simulink model "Exp2"  (R2020a)
settings: Solver=VariableStepAuto  StartTime=0.0  StopTime=25  RelTol=1e-3
InitFcn:
  | Voc=32.9;
  | Iscn=8.21;
  | k=1.38e-23;
  | Ns=54;
  | Np=1;
  | G=800;
  | Gn=1000;
  | Kv=-0.1230;
  | KI=0.0032;
  | T=301;
  | Tn=300;
  | q=1.6e-19;
  | n=1;
  | I0n=9.85e-8;
  | Eg=1.12;
  | Ign=8.214;
  | Rs=0.221;
  | Rp=414.5;
  | a=1.0
libraries: powerlib x7, simulink x1
settings Model: Creator=ahmed  LastModifiedBy=ahmed
settings DataIOCC: Refine=250

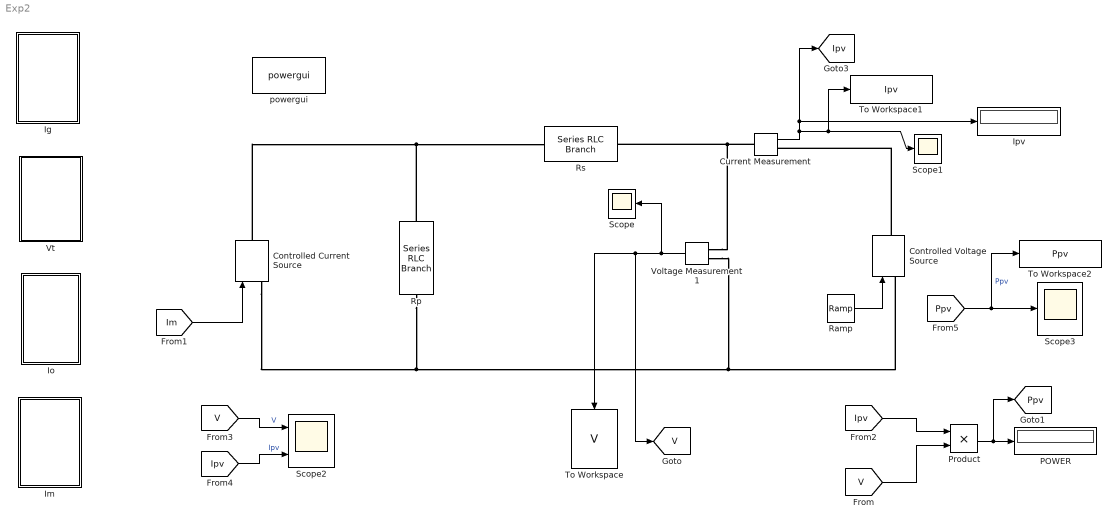
== system Exp2 ==
  Controlled Current Source : powerlib/Electrical Sources/Controlled Current Source  Initialize=on  Source_Type=AC  Amplitude=0  Phase=0  Frequency=0  Measurements=None
  Controlled Voltage Source : powerlib/Electrical Sources/Controlled Voltage Source  Initialize=on  Source_Type=AC  Amplitude=0  Phase=0  Frequency=0  Measurements=None
  Current Measurement : powerlib/Measurements/Current Measurement  PhasorSimulation=off  OutputType=Complex  PSBequivalent=0
  Ig : Subsystem
  Im : Subsystem
  Io : Subsystem
  Ipv : Display
  POWER : Display
  Product : Product
  Ramp : simulink/Sources/Ramp  slope=1  start=0  InitialOutput=0
  Rp : powerlib/Elements/Series RLC Branch  LConnTagsString=__new0  RConnTagsString=__new0  BranchType=R  Resistance=Rp  Inductance=1e-3  SetiL0=off  InitialCurrent=0  Capacitance=1e-6  Setx0=off  InitialVoltage=0  Measurements=None
  Rs : powerlib/Elements/Series RLC Branch  LConnTagsString=__new0  RConnTagsString=__new0  BranchType=R  Resistance=Rs  Inductance=1e-3  SetiL0=off  InitialCurrent=0  Capacitance=1e-6  Setx0=off  InitialVoltage=0  Measurements=None
  Scope : Scope
  Scope1 : Scope
  Scope2 : Scope  NumInputPorts=2
  Scope3 : Scope
  To Workspace : ToWorkspace  VariableName=V  SaveFormat=Timeseries  SampleTime=-1
  To Workspace1 : ToWorkspace  VariableName=Ipv  SaveFormat=Timeseries  SampleTime=-1
  To Workspace2 : ToWorkspace  VariableName=Ppv  SaveFormat=Timeseries  SampleTime=-1
  Voltage Measurement1 : powerlib/Measurements/Voltage Measurement  PhasorSimulation=off  OutputType=Complex  PSBequivalent=0
  Vt : Subsystem
  powergui : powerlib/powergui  Priority=1  SimulationMode=Continuous  SampleTime=50e-6  frequency=60  Iterations=50  frequencyindice=0  Pbase=100e6  ErrMax=1e-4  UnitsV=kV  UnitsW=MW  buscounter=0  FunctionMessages=off  echomessages=off  EnableUseOfTLC=off  CurrentSourceSwitches=off  DisableSnubberDevices=off  DisableRonSwitches=off  DisableVfSwitches=off  DisplayEquations=off  AutomaticDiscreteSolvers=off  SolverType=Tustin/Backward Euler (TBE)  Interpol=off  ExternalGateDelay=off  methode=off  Ts=100  x0status=blocks  SPID=on  SwTol=0  HookPort=off  NonlinearTolerance=1e-4  nMaxIteration=100  ContinueOnMaxIteration=off  RestoreLinks=warning  ResistiveCurrentMeasurement=off  Frange=[0:2:500]  Ylog=off  Xlog=on  ShowGrid=off  save=off  variable=ZData  structure=0  ZoomFFT=off  StartTime=0.0  cycles=1  DisplayStyle=1  fundamental=60  FreqAxis=off  MaxFrequency=1000  frequencyindicesteady=1  RmsSteady=1  display=off
  tag scope: Ipv=global, Ppv=global, V=global
  wires:
  [Im] -> Controlled Current Source/1
  Ramp/1 -> Controlled Voltage Source/1
  Voltage Measurement1/1 -> [V], To Workspace/1, Scope/1
  [Ipv] -> Product/1
  [V] -> Product/2
  Product/1 -> [Ppv], POWER/1
  [V] -> Scope2/1  "V"
  [Ipv] -> Scope2/2  "Ipv"
  [Ppv] -> To Workspace2/1, Scope3/1  "Ppv"
  Current Measurement/1 -> Scope1/1, To Workspace1/1, Ipv/1, [Ipv]
  connections:
  Controlled Current Source/RConn1 -- Rs/LConn1 -- Rp/LConn1
  Current Measurement/LConn1 -- Voltage Measurement1/LConn1 -- Rs/RConn1
  Controlled Voltage Source/RConn1 -- Current Measurement/RConn1
  Controlled Current Source/LConn1 -- Voltage Measurement1/LConn2 -- Controlled Voltage Source/LConn1 -- Rp/RConn1

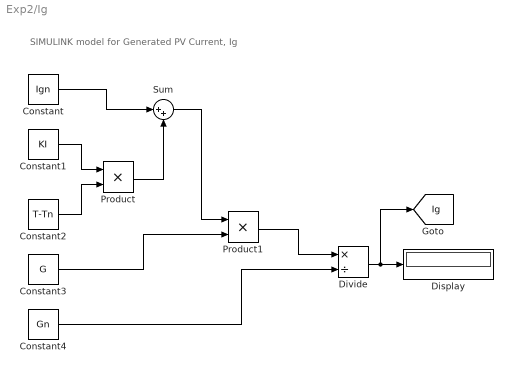
== system Exp2/Ig ==
  note: SIMULINK model for Generated PV Current, Ig
  Constant : Constant  Value=Ign
  Constant1 : Constant  Value=KI
  Constant2 : Constant  Value=T-Tn
  Constant3 : Constant  Value=G
  Constant4 : Constant  Value=Gn
  Display : Display
  Divide : Product  Inputs=*/
  Product : Product
  Product1 : Product
  Sum : Sum  Inputs=|++
  tag scope: Ig=global
  wires:
  Divide/1 -> [Ig], Display/1
  Product1/1 -> Divide/1
  Constant1/1 -> Product/1
  Constant/1 -> Sum/1
  Product/1 -> Sum/2
  Constant2/1 -> Product/2
  Constant3/1 -> Product1/2
  Sum/1 -> Product1/1
  Constant4/1 -> Divide/2

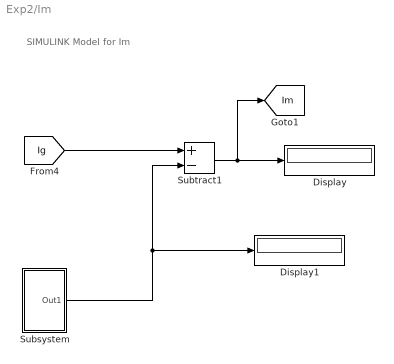
== system Exp2/Im ==
  note: SIMULINK Model for Im
  Display : Display
  Display1 : Display
  Subsystem : Subsystem
  Subtract1 : Sum  Inputs=+-
  tag scope: Im=global
  wires:
  [Ig] -> Subtract1/1
  Subtract1/1 -> [Im], Display/1
  Subsystem/1(Out1) -> Display1/1, Subtract1/2

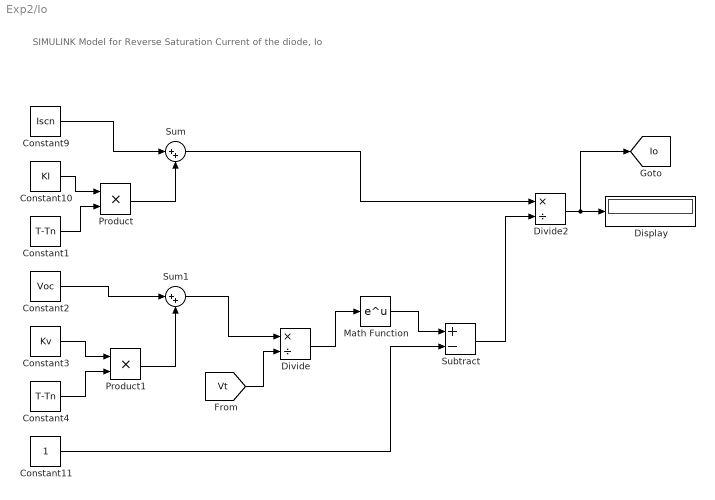
== system Exp2/Io ==
  note: SIMULINK Model for Reverse Saturation Current of the diode, Io
  Constant1 : Constant  Value=T-Tn
  Constant10 : Constant  Value=KI
  Constant11 : Constant
  Constant2 : Constant  Value=Voc
  Constant3 : Constant  Value=Kv
  Constant4 : Constant  Value=T-Tn
  Constant9 : Constant  Value=Iscn
  Display : Display
  Divide : Product  Inputs=*/
  Divide2 : Product  Inputs=*/
  Math Function : Math  SaturateOnIntegerOverflow=on
  Product : Product
  Product1 : Product
  Subtract : Sum  Inputs=+-
  Sum : Sum  Inputs=|++
  Sum1 : Sum  Inputs=|++
  tag scope: Io=global
  wires:
  Constant4/1 -> Product1/2
  [Vt] -> Divide/2
  Product/1 -> Sum/2
  Math Function/1 -> Subtract/1
  Sum/1 -> Divide2/1
  Constant9/1 -> Sum/1
  Product1/1 -> Sum1/2
  Constant11/1 -> Subtract/2
  Constant3/1 -> Product1/1
  Sum1/1 -> Divide/1
  Divide2/1 -> [Io], Display/1
  Constant10/1 -> Product/1
  Subtract/1 -> Divide2/2
  Constant2/1 -> Sum1/1
  Divide/1 -> Math Function/1
  Constant1/1 -> Product/2

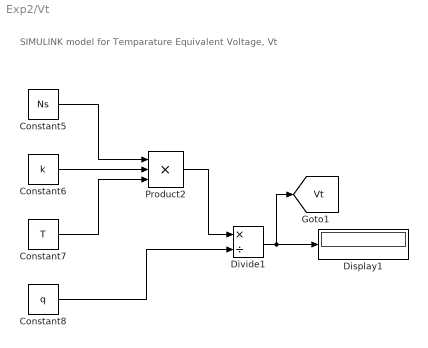
== system Exp2/Vt ==
  note: SIMULINK model for Temparature Equivalent Voltage, Vt
  Constant5 : Constant  Value=Ns
  Constant6 : Constant  Value=k
  Constant7 : Constant  Value=T
  Constant8 : Constant  Value=q
  Display1 : Display
  Divide1 : Product  Inputs=*/
  Product2 : Product  Inputs=3
  tag scope: Vt=global
  wires:
  Product2/1 -> Divide1/1
  Divide1/1 -> [Vt], Display1/1
  Constant5/1 -> Product2/1
  Constant7/1 -> Product2/3
  Constant8/1 -> Divide1/2
  Constant6/1 -> Product2/2

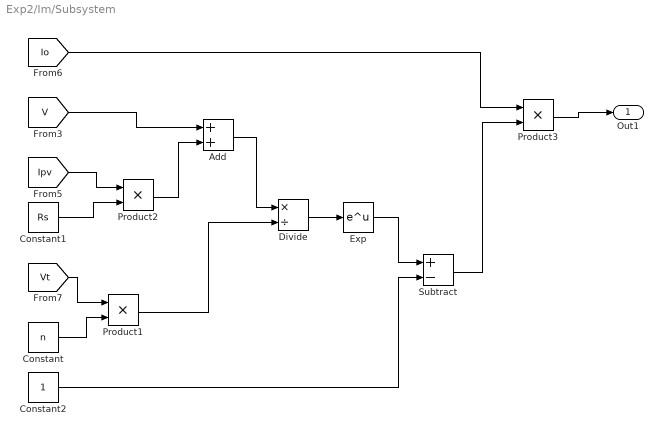
== system Exp2/Im/Subsystem ==
  Add : Sum
  Constant : Constant  Value=n
  Constant1 : Constant  Value=Rs
  Constant2 : Constant
  Divide : Product  Inputs=*/
  Exp : Math  SaturateOnIntegerOverflow=on
  Product1 : Product
  Product2 : Product
  Product3 : Product
  Subtract : Sum  Inputs=+-
  Out1 : Outport
  wires:
  Product2/1 -> Add/2
  Divide/1 -> Exp/1
  [Ipv] -> Product2/1
  [Vt] -> Product1/1
  Constant1/1 -> Product2/2
  [Io] -> Product3/1
  Add/1 -> Divide/1
  Constant2/1 -> Subtract/2
  Product1/1 -> Divide/2
  Exp/1 -> Subtract/1
  Subtract/1 -> Product3/2
  Constant/1 -> Product1/2
  [V] -> Add/1
  Product3/1 -> Out1/1
